simulink model "Bremsvorgang"  (R2023a)
settings: Solver=VariableStepAuto  StartTime=0.0  StopTime=10.0  RelTol=1e-3
libraries: simulink x2
settings Model: Creator=victoriastrobel  LastModifiedBy=tinah

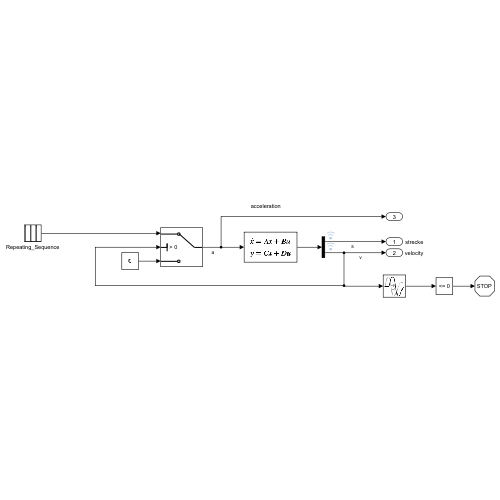
[thumbnail: Simulink's stored preview of the top-level diagram]
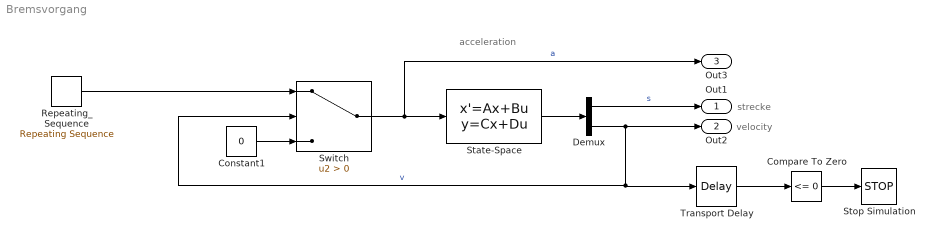
== system Bremsvorgang ==
  note: acceleration
  note: velocity
  note: strecke
  Compare To Zero : simulink/Logic and Bit Operations/Compare To Zero  relop=<=  OutDataTypeStr=boolean
  Constant1 : Constant  Value=0
  Demux : Demux  Outputs=2
  Repeating_Sequence : simulink/Sources/Repeating Sequence  rep_seq_t=repeating_sequence  rep_seq_y=repeating_sequence_out
  State-Space : StateSpace  A=[0 1; 0 0]  B=[0; 1]  C=[1 0; 0 1]  D=[0; 0]  InitialCondition=[10, 10]
  Stop Simulation : Stop
  Switch : Switch  Criteria=u2 > Threshold  SaturateOnIntegerOverflow=off  InputSameDT=off
  Transport Delay : TransportDelay  InitialOutput=1
  Out1 : Outport
  Out2 : Outport  Port=2
  Out3 : Outport  Port=3
  wires:
  State-Space/1 -> Demux/1
  Demux/1 -> Out1/1  "s"
  Demux/2 -> Transport Delay/1, Switch/2, Out2/1  "v"
  Switch/1 -> Out3/1, State-Space/1  "a"
  Constant1/1 -> Switch/3
  Transport Delay/1 -> Compare To Zero/1
  Compare To Zero/1 -> Stop Simulation/1
  Repeating_Sequence/1 -> Switch/1
